simulink model "Fig57"  (R2014b)
settings: Solver=ode3  StartTime=0.0  StopTime=1.048576  FixedStep=2e-6  RelTol=1e-5
libraries: commrandsrc2 x3, commanapbnd3 x2, commchan3 x1
settings Model: Creator=Dennis Silage  LastModifiedBy=Silage
settings DataIOCC: SignalLoggingSaveFormat=ModelDataLogs
settings OptimizationCC: ExpressionDepthLimit=2147483647  InitFltsAndDblsToZero=on
settings DebuggingCC: UnderspecifiedInitializationDetection=Classic  MergeDetectMultiDrivingBlocksExec=none  SolverPrmCheckMsg=none  FcnCallInpInsideContextMsg=UseLocalSettings  StateNameClashWarn=warning
settings GRTTargetCC: CombineOutputUpdateFcns=off  GRTInterface=on

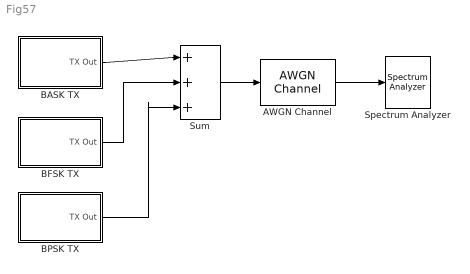
== system Fig57 ==
  AWGN Channel : commchan3/AWGN Channel  InputProcessing=Inherited (this choice will be removed - see release notes)  seed=randseed  noiseMode="Signal to noise ratio  (Eb/No)"  EbNodB=80  EsNodB=10  SNRdB=12  bitsPerSym=1  Ps=12.5  Tsym=1e-3  variance=0
  BASK TX : Subsystem
  BFSK TX : Subsystem
  BPSK TX : Subsystem
  Spectrum Analyzer : SpectrumAnalyzer
  Sum : Sum  Inputs=|+|+|+|
  wires:
  BASK TX/1(TX Out) -> Sum/1
  BFSK TX/1(TX Out) -> Sum/2
  BPSK TX/1(TX Out) -> Sum/3
  Sum/1 -> AWGN Channel/1
  AWGN Channel/1 -> Spectrum Analyzer/1

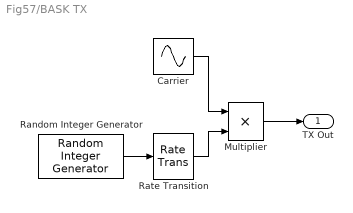
== system Fig57/BASK TX ==
  Carrier : Sin  Amplitude=5  Frequency=31000*pi  SampleTime=2e-6
  "Multiplier " : Product  RndMeth=Zero
  Random Integer Generator : commrandsrc2/Random Integer Generator  mul=2  seed=randseed  Ts=1e-3  frameBased=off  sampPerFrame=50  orient=on  outDataType=double
  Rate Transition : RateTransition  OutPortSampleTime=2e-6
  TX Out : Outport
  wires:
  Random Integer Generator/1 -> Rate Transition/1
  "Multiplier "/1 -> TX Out/1
  Carrier/1 -> "Multiplier "/1
  Rate Transition/1 -> "Multiplier "/2

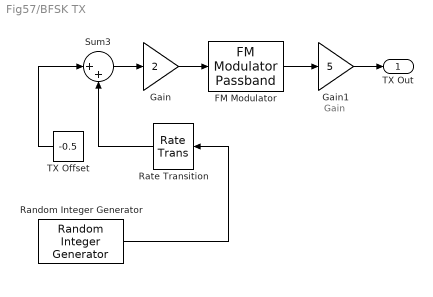
== system Fig57/BFSK TX ==
  note: Gain
  FM Modulator : commanapbnd3/FM Modulator Passband  Fc=20000  Ph=0  Kc=500
  Gain : Gain  Gain=2
  Gain1 : Gain  Gain=5
  Random Integer Generator : commrandsrc2/Random Integer Generator  mul=2  seed=46  Ts=1e-3  frameBased=off  sampPerFrame=50  orient=on  outDataType=double
  Rate Transition : RateTransition  OutPortSampleTime=2e-6
  Sum3 : Sum  Inputs=|++
  TX Offset : Constant  Value=-0.5
  TX Out : Outport
  wires:
  Sum3/1 -> Gain/1
  TX Offset/1 -> Sum3/1
  Random Integer Generator/1 -> Rate Transition/1
  Rate Transition/1 -> Sum3/2
  Gain/1 -> FM Modulator/1
  FM Modulator/1 -> Gain1/1
  Gain1/1 -> TX Out/1

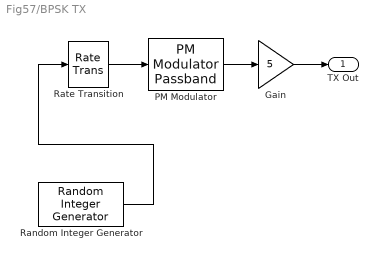
== system Fig57/BPSK TX ==
  Gain : Gain  Gain=5
  PM Modulator : commanapbnd3/PM Modulator Passband  Fc=24500  Ph=pi  Kc=pi
  Random Integer Generator : commrandsrc2/Random Integer Generator  mul=2  seed=randseed  Ts=1e-3  frameBased=off  sampPerFrame=50  orient=on  outDataType=double
  Rate Transition : RateTransition  OutPortSampleTime=2e-6
  TX Out : Outport
  wires:
  PM Modulator/1 -> Gain/1
  Rate Transition/1 -> PM Modulator/1
  Gain/1 -> TX Out/1
  Random Integer Generator/1 -> Rate Transition/1
